simulink library "Powernet"  (R2016a)
settings: Solver=ode45  StartTime=0.0  StopTime=10.0  RelTol=1e-3
undefined symbols (not defined in the file): aux_power_selector_aux_power_flag
settings Model: Creator=krishs1  LastModifiedBy=krishs1
settings DataIOCC: LimitDataPoints=on
settings DebuggingCC: AllowSymbolicDim=off

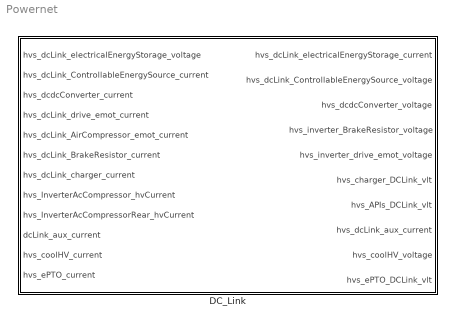
== system Powernet ==
  DC_Link : Subsystem

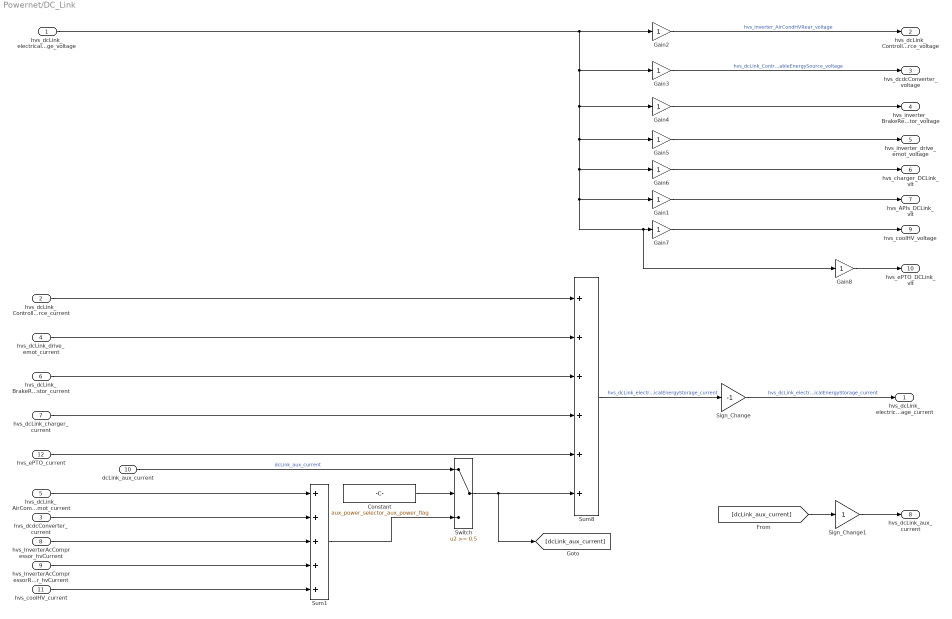
== system Powernet/DC_Link ==
  hvs_dcLink_electricalEnergyStorage_voltage : Inport
  hvs_dcLink_ControllableEnergySource_current : Inport  Port=2
  hvs_dcdcConverter_current : Inport  Port=3
  hvs_dcLink_drive_emot_current : Inport  Port=4
  hvs_dcLink_AirCompressor_emot_current : Inport  Port=5
  hvs_dcLink_BrakeResistor_current : Inport  Port=6
  hvs_dcLink_charger_current : Inport  Port=7
  hvs_InverterAcCompressor_hvCurrent : Inport  Port=8
  hvs_InverterAcCompressorRear_hvCurrent : Inport  Port=9
  dcLink_aux_current : Inport  Port=10
  hvs_coolHV_current : Inport  Port=11
  hvs_ePTO_current : Inport  Port=12
  Constant : Constant  Value=aux_power_selector_aux_power_flag
  Gain{1..8} (8 alike) : Gain
  Sign_Change : Gain  Gain=-1
      mask init:
      | K = str2num(get_param(bdroot,'FixedStep'));
  Sign_Change1 : Gain
      mask init:
      | K = str2num(get_param(bdroot,'FixedStep'));
  Sum1 : Sum  Inputs=+++++  SaturateOnIntegerOverflow=on  InputSameDT=on  OutDataTypeStr=Inherit: Same as first input
  Sum8 : Sum  Inputs=++++++  SaturateOnIntegerOverflow=on  InputSameDT=on  OutDataTypeStr=Inherit: Same as first input
  Switch : Switch  Threshold=0.5
  hvs_dcLink_electricalEnergyStorage_current : Outport
  hvs_dcLink_ControllableEnergySource_voltage : Outport  Port=2
  hvs_dcdcConverter_voltage : Outport  Port=3
  hvs_inverter_BrakeResistor_voltage : Outport  Port=4
  hvs_inverter_drive_emot_voltage : Outport  Port=5
  hvs_charger_DCLink_vlt : Outport  Port=6
  hvs_APIs_DCLink_vlt : Outport  Port=7
  hvs_dcLink_aux_current : Outport  Port=8
  hvs_coolHV_voltage : Outport  Port=9
  hvs_ePTO_DCLink_vlt : Outport  Port=10
  wires:
  hvs_ePTO_current/1 -> Sum8/5
  Gain8/1 -> hvs_ePTO_DCLink_vlt/1
  Gain1/1 -> hvs_APIs_DCLink_vlt/1
  Sign_Change/1 -> hvs_dcLink_electricalEnergyStorage_current/1  "hvs_dcLink_electricalEnergyStorage_current"
  hvs_dcLink_electricalEnergyStorage_voltage/1 -> Gain6/1, Gain7/1, Gain8/1, Gain1/1, Gain5/1, Gain4/1, Gain3/1, Gain2/1
  Gain2/1 -> hvs_dcLink_ControllableEnergySource_voltage/1  "hvs_inverter_AirCondHVRear_voltage"
  Gain3/1 -> hvs_dcdcConverter_voltage/1  "hvs_dcLink_ControllableEnergySource_voltage"
  hvs_dcLink_drive_emot_current/1 -> Sum8/2
  hvs_dcLink_AirCompressor_emot_current/1 -> Sum1/1
  hvs_dcdcConverter_current/1 -> Sum1/2
  Gain4/1 -> hvs_inverter_BrakeResistor_voltage/1
  Gain5/1 -> hvs_inverter_drive_emot_voltage/1
  hvs_dcLink_ControllableEnergySource_current/1 -> Sum8/1
  hvs_dcLink_BrakeResistor_current/1 -> Sum8/3
  Sum8/1 -> Sign_Change/1  "hvs_dcLink_electricalEnergyStorage_current"
  Gain6/1 -> hvs_charger_DCLink_vlt/1
  hvs_InverterAcCompressor_hvCurrent/1 -> Sum1/3
  hvs_InverterAcCompressorRear_hvCurrent/1 -> Sum1/4
  Sum1/1 -> Switch/3
  Switch/1 -> Sum8/6, [dcLink_aux_current]
  dcLink_aux_current/1 -> Switch/1  "dcLink_aux_current"
  Constant/1 -> Switch/2
  hvs_dcLink_charger_current/1 -> Sum8/4
  [dcLink_aux_current] -> Sign_Change1/1
  Sign_Change1/1 -> hvs_dcLink_aux_current/1
  hvs_coolHV_current/1 -> Sum1/5
  Gain7/1 -> hvs_coolHV_voltage/1
